simulink subsystem "NoBMS"  (R2024a)
settings: Solver=VariableStepAuto  StartTime=0.0  StopTime=10.0  RelTol=1e-3
undefined symbols (not defined in the file): CurrentLimitsBus
settings Model: ModifiedByFormat=The MathWorks, Inc.  Creator=The MathWorks, Inc.  LastModifiedBy=The MathWorks, Inc.
settings RTWCC: GPUComputeCapability=3.5

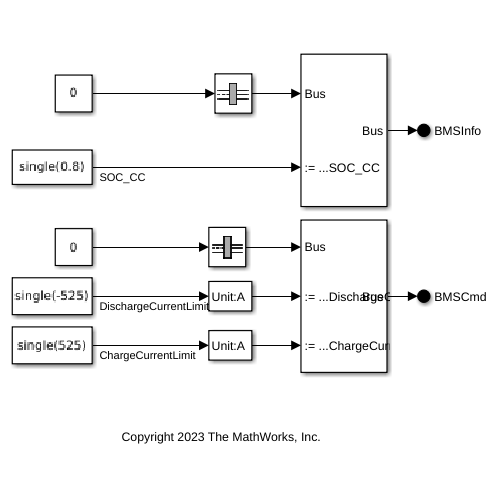
[thumbnail: Simulink's stored preview of the top-level diagram]
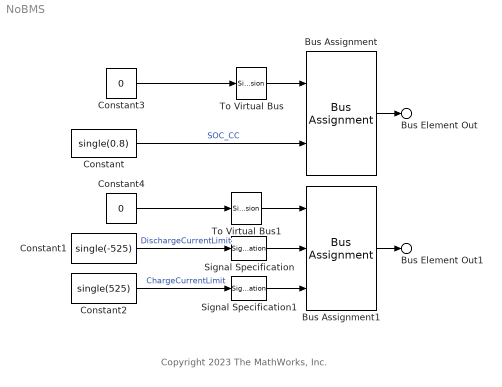
== system NoBMS ==
  note: Copyright 2023 The MathWorks, Inc.
  Bus Assignment : BusAssignment  AssignedSignals=SOC.SOC_CC
  Bus Assignment1 : BusAssignment  AssignedSignals=CurrentLimitsBus.DischargeCurrentLimit,CurrentLimitsBus.ChargeCurrentLimit
  Constant : Constant  Value=single(0.8)  SampleTime=-1
  Constant1 : Constant  Value=single(-525)  SampleTime=-1
  Constant2 : Constant  Value=single(525)  SampleTime=-1
  Constant3 : Constant  Value=0  OutDataTypeStr=Bus: BMSInfoBUS  SampleTime=Inf
  Constant4 : Constant  Value=0  OutDataTypeStr=Bus: BMSCmdBUS  SampleTime=Inf
  Signal Specification : SignalSpecification  Unit=A
  Signal Specification1 : SignalSpecification  Unit=A
  To Virtual Bus : SignalConversion  ConversionOutput=Virtual bus  OverrideOpt=off
  To Virtual Bus1 : SignalConversion  ConversionOutput=Virtual bus  OverrideOpt=off
  Bus Element Out : Outport  PortName=BMSInfo
  Bus Element Out1 : Outport  Port=2  PortName=BMSCmd
  wires:
  Constant/1 -> Bus Assignment/2  "SOC_CC"
  Constant1/1 -> Signal Specification/1  "DischargeCurrentLimit"
  Constant2/1 -> Signal Specification1/1  "ChargeCurrentLimit"
  Signal Specification1/1 -> Bus Assignment1/3
  Constant3/1 -> To Virtual Bus/1
  To Virtual Bus/1 -> Bus Assignment/1
  Bus Assignment/1 -> Bus Element Out/1
  To Virtual Bus1/1 -> Bus Assignment1/1
  Constant4/1 -> To Virtual Bus1/1
  Signal Specification/1 -> Bus Assignment1/2
  Bus Assignment1/1 -> Bus Element Out1/1
